simulink model "MovingObstacleAvoidanceMPC"  (R2018b)
settings: Solver=VariableStepAuto  StartTime=0.0  StopTime=10.0  RelTol=1e-3
values from neighbouring files (symbols this model uses):
  car = struct    [main_one_obstacle.m]
  obstacle = obstacleGenerateObstacleGeometryInfo(obstacle)    [main_one_obstacle.m]
  ref = [0 0 0 car.V]    [main_one_obstacle.m]
  road = struct    [main_one_obstacle.m]
libraries: mpclib x1
settings Model: Creator=alberto  LastModifiedBy=alberto

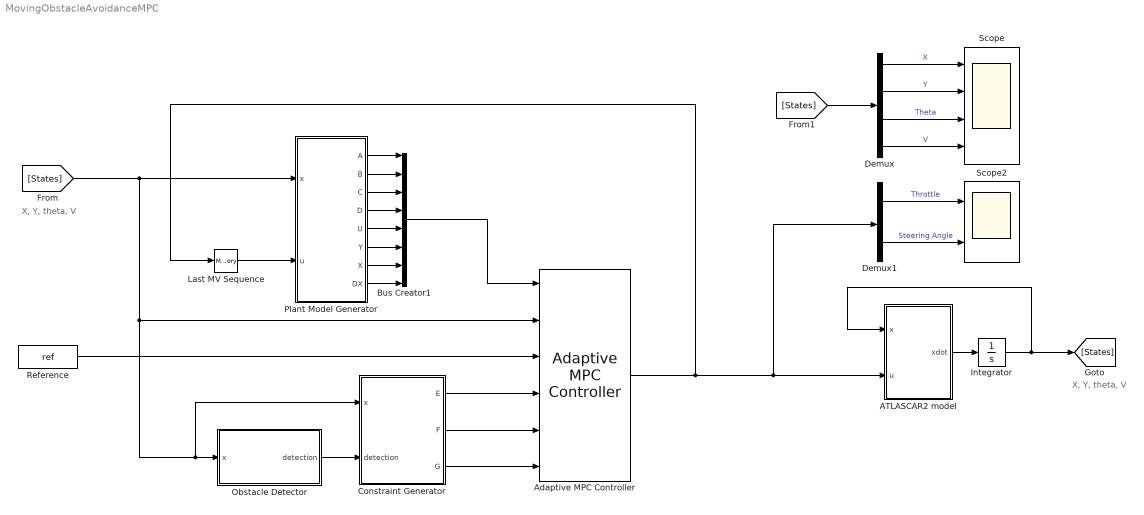
== system MovingObstacleAvoidanceMPC ==
  note: X, Y, theta, V
  note: X, Y, theta, V
  ATLASCAR2 model : MATLAB Function  TreatAsAtomicUnit=on
  Adaptive MPC Controller : mpclib/Adaptive MPC Controller  SCDEnableBlockLinearizationSpecification=on  mpcobj=mpcobj  enable_value=0  updateMPCinCallerWorkspace=on  md_inport=off  mv_inport=off  return_cost=off  return_mvseq=off  return_qpstatus=off  return_xseq=off  return_state=off  return_ovseq=off  state_inport=off  isltv_plant=off  umin_inport=off  umax_inport=off  ymin_inport=off  ymax_inport=off  cc_inport=on  ywt_inport=off  uwt_inport=off  duwt_inport=off  rhoeps_inport=off  uref_inport=off  BlockDataType=double  SampleTimeInherited=off  switch_inport=off
      settings: SourceProductName=Model Predictive Control Toolbox
  Bus Creator1 : BusCreator  Inputs=8
  Constraint Generator : MATLAB Function  TreatAsAtomicUnit=on
  Demux : Demux
  Demux1 : Demux  Outputs=2
  Integrator : Integrator  InitialCondition=car.x0
  Last MV Sequence : Memory  InitialCondition=car.u0  InheritSampleTime=on
  Obstacle Detector : MATLAB Function  TreatAsAtomicUnit=on
  Plant Model Generator : MATLAB Function  TreatAsAtomicUnit=on
  Reference : Constant  Value=ref
  Scope : Scope  NumInputPorts=4
  Scope2 : Scope  NumInputPorts=2
  wires:
  Bus Creator1/1 -> Adaptive MPC Controller/1
  Constraint Generator/1(E) -> Adaptive MPC Controller/4
  ATLASCAR2 model/1(xdot) -> Integrator/1
  [States] -> Adaptive MPC Controller/2, Obstacle Detector/1(x), Constraint Generator/1(x), Plant Model Generator/1(x)
  Constraint Generator/3(G) -> Adaptive MPC Controller/6
  Plant Model Generator/8(DX) -> Bus Creator1/8
  Last MV Sequence/1 -> Plant Model Generator/2(u)
  Reference/1 -> Adaptive MPC Controller/3
  Plant Model Generator/3(C) -> Bus Creator1/3
  Integrator/1 -> [States], ATLASCAR2 model/1(x)
  Plant Model Generator/4(D) -> Bus Creator1/4
  Demux/4 -> Scope/4  "V"
  Plant Model Generator/1(A) -> Bus Creator1/1
  Demux/1 -> Scope/1  "X"
  Plant Model Generator/2(B) -> Bus Creator1/2
  Demux/3 -> Scope/3  "Theta"
  Plant Model Generator/6(Y) -> Bus Creator1/6
  Plant Model Generator/7(X) -> Bus Creator1/7
  Adaptive MPC Controller/1 -> Last MV Sequence/1, Demux1/1, ATLASCAR2 model/2(u)
  Demux/2 -> Scope/2  "Y"
  Constraint Generator/2(F) -> Adaptive MPC Controller/5
  Plant Model Generator/5(U) -> Bus Creator1/5
  Obstacle Detector/1(detection) -> Constraint Generator/2(detection)
  Demux1/1 -> Scope2/1  "Throttle"
  [States] -> Demux/1
  Demux1/2 -> Scope2/2  "Steering Angle"

== matlab function MovingObstacleAvoidanceMPC/ATLASCAR2 model ==
  settings: updateMethod=DISCRETE  sampleTime=Ts
  data: x input; u input; xdot output
function xdot = fcn(x,u)
xdot = ATLASCAR2ModelCT(x,u);

== matlab function MovingObstacleAvoidanceMPC/Plant Model Generator ==
  settings: updateMethod=DISCRETE  sampleTime=Ts
  data: x input; u input; A output; B output; C output; D output; U output size=[2,1]; Y output size=[4,1]; X output size=[4,1]; DX output size=[4,1]; Ts parameter
function [A,B,C,D,U,Y,X,DX] = fcn(x,u,Ts)
[A,B,C,D,U,Y,X,DX] = ATLASCAR2ModelDT(Ts,x,u);

== matlab function MovingObstacleAvoidanceMPC/Obstacle Detector ==
  settings: updateMethod=DISCRETE  sampleTime=Ts
  data: x input; obstacle parameter; road parameter; detection output
function detection  = fcn(x,obstacle,road)
% Detection Logic: it determine when the vehicle sees the obstacle
detection = obstacleDetect(x,obstacle,road.laneWidth);

== matlab function MovingObstacleAvoidanceMPC/Constraint Generator ==
  settings: updateMethod=DISCRETE  sampleTime=Ts
  data: x input; detection input; obstacle parameter; road parameter; E output; F output; G output
function [E,F,G] = fcn(x,detection,obstacle,road)
% Generate run-time custom constraint
[E,F,G] = obstacleComputeCustomConstraint(x,detection,obstacle,road.laneWidth,road.lanes);
